simulink model "pid_02"  (Simulink 10.0)
settings: Solver=ode3  StartTime=0.0  StopTime=10  RelTol=1e-3
model workspace (MATLAB code in the model file):
  | SampleRate = 20000; % Sample rate
  | Ts = 1/SampleRate;     % System samplerate
  | M = 1.4e-6; % Mass in kg
  | saturationlimit=7.9999; % Saturation in controller
  | % motionprofile configuration
  | acceleration=4000000; % Parameter for stimulus
  | accel_period=10; % Parameter for stimulus
settings Model: FPTRunName=Active  Creator=tjia  LastModifiedBy=bhisma
settings SolverCC: AutoInsertRateTranBlk=on
settings DataIOCC: LimitDataPoints=on  SignalLoggingSaveFormat=ModelDataLogs  SaveOutput=off  SignalLogging=off  DSMLogging=off  SaveTime=off
settings OptimizationCC: BlockReduction=off  ConditionallyExecuteInputs=off  DefaultParameterBehavior=Inlined  ExpressionDepthLimit=2147483647
settings DebuggingCC: AlgebraicLoopMsg=error  SolverPrmCheckMsg=warning  MultiTaskCondExecSysMsg=warning  MultiTaskRateTransMsg=warning  IntegerOverflowMsg=none  ParameterOverflowMsg=warning  ParameterPrecisionLossMsg=none  FcnCallInpInsideContextMsg=warning  StateNameClashWarn=warning  IntegerSaturationMsg=none
settings HardwareCC: ProdHWDeviceType=ASIC/FPGA->ASIC/FPGA  ProdEqTarget=off
settings GRTTargetCC: GeneratePreprocessorConditionals=Disable all
settings ConfigComp: CovExternalEMLEnable=off  CovSFcnEnable=off

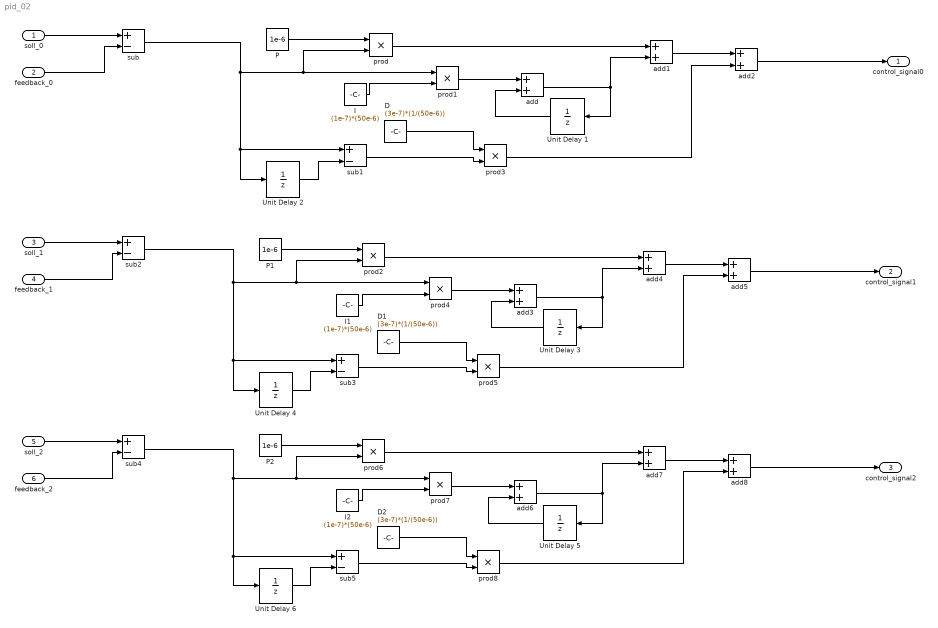
== system pid_02 ==
  soll_0 : Inport  OutDataTypeStr=fixdt(1,32,16)
  feedback_0 : Inport  Port=2  OutDataTypeStr=fixdt(1,32,16)
  soll_1 : Inport  Port=3  OutDataTypeStr=fixdt(1,32,16)
  feedback_1 : Inport  Port=4  OutDataTypeStr=fixdt(1,32,16)
  soll_2 : Inport  Port=5  OutDataTypeStr=fixdt(1,32,16)
  feedback_2 : Inport  Port=6  OutDataTypeStr=fixdt(1,32,16)
  D : Constant  Value=(3e-7)*(1/(50e-6))  OutDataTypeStr=Inherit: Inherit via back propagation
  D1 : Constant  Value=(3e-7)*(1/(50e-6))  OutDataTypeStr=Inherit: Inherit via back propagation
  D2 : Constant  Value=(3e-7)*(1/(50e-6))  OutDataTypeStr=Inherit: Inherit via back propagation
  I : Constant  Value=(1e-7)*(50e-6)  OutDataTypeStr=fixdt(1,16,34)
  I1 : Constant  Value=(1e-7)*(50e-6)  OutDataTypeStr=fixdt(1,16,34)
  I2 : Constant  Value=(1e-7)*(50e-6)  OutDataTypeStr=fixdt(1,16,34)
  P : Constant  Value=1e-6  OutDataTypeStr=fixdt(1,16,34)
  P1 : Constant  Value=1e-6  OutDataTypeStr=fixdt(1,16,34)
  P2 : Constant  Value=1e-6  OutDataTypeStr=fixdt(1,16,34)
  Unit Delay {1..6} (6 alike) : UnitDelay  SampleTime=-1  HasFrameUpgradeWarning=on
  add{,1..8} (9 alike) : Sum  OutDataTypeStr=fixdt(1,32,28)
  prod{,1..8} (9 alike) : Product  OutDataTypeStr=fixdt(1,32,33)  RndMeth=Zero
  sub{,1..5} (6 alike) : Sum  Inputs=+-  OutDataTypeStr=fixdt(1,32,16)
  control_signal0 : Outport
  control_signal1 : Outport  Port=2
  control_signal2 : Outport  Port=3
  wires:
  P/1 -> prod/1
  add/1 -> Unit Delay 1/1, add1/2
  Unit Delay 1/1 -> add/2
  add1/1 -> add2/1
  add2/1 -> control_signal0/1
  soll_0/1 -> sub/1
  feedback_0/1 -> sub/2
  sub/1 -> prod/2, prod1/1, Unit Delay 2/1, sub1/1
  prod/1 -> add1/1
  prod1/1 -> add/1
  I/1 -> prod1/2
  sub1/1 -> prod3/2
  D/1 -> prod3/1
  prod3/1 -> add2/2
  Unit Delay 2/1 -> sub1/2
  P1/1 -> prod2/1
  add3/1 -> Unit Delay 3/1, add4/2
  Unit Delay 3/1 -> add3/2
  add4/1 -> add5/1
  add5/1 -> control_signal1/1
  soll_1/1 -> sub2/1
  feedback_1/1 -> sub2/2
  sub2/1 -> prod2/2, prod4/1, Unit Delay 4/1, sub3/1
  prod2/1 -> add4/1
  prod4/1 -> add3/1
  I1/1 -> prod4/2
  sub3/1 -> prod5/2
  D1/1 -> prod5/1
  prod5/1 -> add5/2
  Unit Delay 4/1 -> sub3/2
  P2/1 -> prod6/1
  add6/1 -> Unit Delay 5/1, add7/2
  Unit Delay 5/1 -> add6/2
  add7/1 -> add8/1
  add8/1 -> control_signal2/1
  soll_2/1 -> sub4/1
  feedback_2/1 -> sub4/2
  sub4/1 -> prod6/2, prod7/1, Unit Delay 6/1, sub5/1
  prod6/1 -> add7/1
  prod7/1 -> add6/1
  I2/1 -> prod7/2
  sub5/1 -> prod8/2
  D2/1 -> prod8/1
  prod8/1 -> add8/2
  Unit Delay 6/1 -> sub5/2
